simulink model "SIM_SAD_DEMO"  (R2025b)
settings: Solver=ode5  StartTime=0.0  StopTime=2*T  FixedStep=0.1  RelTol=1e-3
model workspace (MAT data in the model file):
  Pnull : Simulink.Parameter (value not decoded)
  rho_albedo_medio : Simulink.Parameter (value not decoded)
values from neighbouring files (symbols this model uses):
  Aree = zeros(10,1)    [SCRIPT_SAD_DEMO.m]
  base_seed = base_seed_MC + k    [SCRIPT_SAD_DEMO.m]
  c = astroConstants(5)*1e3    [SCRIPT_SAD_DEMO.m]
  draan = 1.99096871e-7    (= 1.99096871e-07)    [SCRIPT_SAD_DEMO.m]
  dwell_time = 30    [SCRIPT_SAD_DEMO.m]
  eps_att = deg2rad(0.2)    [SCRIPT_SAD_DEMO.m]
  eps_E = deg2rad(astroConstants(63))    [SCRIPT_SAD_DEMO.m]
  eps_h_r = 0.001    [SCRIPT_SAD_DEMO.m]
  eps_w = deg2rad(0.1)    [SCRIPT_SAD_DEMO.m]
  err_max = deg2rad(15)    [SCRIPT_SAD_DEMO.m]
  F_e = 1358    [SCRIPT_SAD_DEMO.m]
  h_r_max = 0.05    [SCRIPT_SAD_DEMO.m]
  h_r_safe = 0.001    [SCRIPT_SAD_DEMO.m]
  j_B = [0.01; 0.05; 0.01]    [SCRIPT_SAD_DEMO.m]
  J_depl = J_nom    [SCRIPT_SAD_DEMO.m]
  JD0 = juliandate(startTime)    [SCRIPT_SAD_DEMO.m]
  k_b = 200000    [SCRIPT_SAD_DEMO.m]
  Kd = K(:, 1:3)    [SCRIPT_SAD_DEMO.m]
  kep = [a,e,incl,raan,w,theta]    [SCRIPT_SAD_DEMO.m]
  Kp = K(:, 4:6)    [SCRIPT_SAD_DEMO.m]
  mu = astroConstants(13)    [SCRIPT_SAD_DEMO.m]
  n = sqrt( (mu/ (a)^3))    [SCRIPT_SAD_DEMO.m]
  n_sun = 2*pi/T_sun    (= 1.99238499086e-07)    [SCRIPT_SAD_DEMO.m]
  Nmat = [ ... (first row only)    [SCRIPT_SAD_DEMO.m]
  r_sun = 1*AU    [SCRIPT_SAD_DEMO.m]
  Re = astroConstants(23)    [SCRIPT_SAD_DEMO.m]
  rf = [ ... (first row only)    [SCRIPT_SAD_DEMO.m]
  rhod = 0.1*ones(10,1)    [SCRIPT_SAD_DEMO.m]
  rhos = zeros(10,1)    [SCRIPT_SAD_DEMO.m]
  SRP = SRP_nom    [SCRIPT_SAD_DEMO.m]
  theta = 0    [SCRIPT_SAD_DEMO.m]
  w0 = w0_nom    [SCRIPT_SAD_DEMO.m]
  w_enter = Control.w_tumbling    [SCRIPT_SAD_DEMO.m]
  w_enter_2 = Control.w_pointing    [SCRIPT_SAD_DEMO.m]
  w_exit = deg2rad(4)    [SCRIPT_SAD_DEMO.m]
  w_exit_2 = deg2rad(1.5)    [SCRIPT_SAD_DEMO.m]
symbols that are objects in the model workspace (value not decoded): Pnull, rho_albedo_medio
undefined symbols (not defined in the file or in its folder): DiscIntNeverNeededParam, Filter, Gyro, Magmeter, MTQ, q, RW, Sun_sensor
libraries: matrix_library x41, LIBRARY_SAD x40, simulink x1, cstblocks x1
(part 4 of 4)

== matlab function SIM_SAD_DEMO/ATTITUDE DETERMINATION (q-method)/MATLAB Function ==
  data: u input; q output
function q = fcn(u)
% u: matrice K del q-method
% q: quaternione "continuo" (ambiguità di segno risolta)

persistent q_prev   % memorizza il quaternione del passo precedente

% 1) autovettore corrispondente all'autovalore massimo
[qvec, D] = eig(u);
[~, n] = max(real(diag(D)));
q = real(qvec(:, n));

% 2) normalizzo
q = q ./ norm(q);

% 3) se è la prima chiamata, non posso confrontare col passato
if isempty(q_prev)
    q_prev = q;
    return;
end

% 4) prodotto scalare col quaternione precedente
val = dot(q, q_prev);

% 5) se cambia ramo, flippa il segno
if val < 0
    q = -q;
end

% 6) aggiorna memoria
q_prev = q;
end

== matlab function SIM_SAD_DEMO/DKE/Magnetic Torque/IGRF magnetic torque/MATLAB Function1 ==
  data: r_ecef input; lat output; lon output
function [lat, lon] = ecef2latlon(r_ecef)
    x = r_ecef(1); y = r_ecef(2); z = r_ecef(3);
    lon = atan2(y, x);
    lat = atan2(z, sqrt(x^2 + y^2));
    lat = rad2deg(lat);
    lon = rad2deg(lon);
end

== matlab function SIM_SAD_DEMO/DKE/Magnetic Torque/IGRF magnetic torque/MATLAB Function2 ==
  data: B_NED input; B_ECI output; lat_deg input; lon_deg input; t input; alpha_G0 input
function B_ECI = ned2eci(B_NED, lat_deg, lon_deg, t,alpha_G0)
    % Converts magnetic field from NED frame to ECI frame
    % Inputs:
    %   B_NED   : [Bx, By, Bz] in NED frame (Tesla or Gauss)
    %   lat_deg : latitude in degrees
    %   lon_deg : longitude in degrees
    %   t       : simulation time in seconds (since reference epoch)
    %
    % Output:
    %   B_ECI   : magnetic field in ECI frame
    
    % Convert degrees to radians
    lat = deg2rad(lat_deg);
    lon = deg2rad(lon_deg);
    
    % Earth rotation rate (rad/s)
    omega_earth = 7.2921159e-5;
    
    % Earth rotation angle since reference epoch (1 Jan 2025)
    theta = alpha_G0 + omega_earth * t;
    
    % --- Step 1: NED → ECEF rotation matrix ---
    R_NED2ECEF = [-sin(lat)*cos(lon), -sin(lon),  -cos(lat)*cos(lon);
                  -sin(lat)*sin(lon), cos(lon),   -cos(lat)*sin(lon);
                  cos(lat),             0,        -sin(lat)];
    
    % Convert B_NED to ECEF
    B_ECEF = R_NED2ECEF * B_NED(:);
    
    % --- Step 2: ECEF → ECI rotation matrix ---
    R_ECEF2ECI = [cos(theta), -sin(theta), 0;
                  sin(theta),  cos(theta), 0;
                  0,           0,          1];
    
    % Convert B_ECEF to ECI
    B_ECI = R_ECEF2ECI * B_ECEF * 1e-9;
end

== stateflow chart SIM_SAD_DEMO/CONTROL/Chart ==
  state DETUMBLING
    during:
    mode = 1;
  state TRACKING
    during:
    mode = 2;
  state RW_DESATURATION
    during:
    mode = 4;
  state POINTING
    during:
    mode = 3;
  (default) -> DETUMBLING
  DETUMBLING -> TRACKING : after(dwell_time, sec) [ norm_w < (w_enter - eps_w) ]
  TRACKING -> DETUMBLING [order 1] : after(dwell_time, sec)[norm_w > (w_exit + eps_w) ]
  POINTING -> TRACKING [order 1] : after(dwell_time, sec)[ (norm_w > (w_exit_2 + eps_w)) || (err_att_track > (err_max + eps_att)) ]
  TRACKING -> POINTING [order 2] : after(dwell_time, sec) [(norm_w < (w_enter_2 - eps_w)) && (err_att_slew < (err_max - eps_att))]
  POINTING -> RW_DESATURATION [order 2] : after(dwell_time, sec)[abs(h_r_feed) > 0.8*(h_r_max-eps_h_r) ]
  RW_DESATURATION -> POINTING : after(dwell_time, sec)[abs(h_r_feed) < h_r_safe ]
  data: norm_w input double size=[1 1]; mode output double size=[1 1]; w_enter parameter; w_exit parameter; w_enter_2 parameter; w_exit_2 parameter; err_att_slew input; eps_w parameter; dwell_time parameter; eps_att parameter; err_max parameter; err_att_track input; h_r_feed input; h_r_safe parameter; h_r_max parameter; eps_h_r parameter
